simulink model "new_nncontroller_5_50"  (R2021a)
settings: Solver=VariableStepAuto  StartTime=0.0  StopTime=10.0  RelTol=1e-3
libraries: neural x257
(part 14 of 14)

== system new_nncontroller_5_50/Feed-Forward Neural Network/Layer 6/Delays 1 ==
  "p{6}" : Inport  PortDimensions=50
      mask Display: e = 0.06;c1 = [120 230 180]/255;c2 = ([120 230 180]+0)/(256+128);c3 = ([120 230 180]+128)/(256+128);patch([0 1 1 0],[0 0 1 1],c1);patch([0 1 1 1-e 1-e 0+e],[0 0 1 1-e 0+e 0+e],c2);patch([0 0 1 1-e 0+e 0+e],[0 1 1 1-e 1-e 0+e],c3);plot([0 1 1 0 0],[0 0 1 1 0]);
  mux : Mux  Inputs=1
      mask Display: e = 0.06;c1 = [120 150 230]/255;c2 = ([120 150 230]+0)/383;c3 = ([120 150 230]+128)/383;patch([0 1 1 0],[0 0 1 1],c1);patch([0 1 1 1-e 1-e 0+e],[0 0 1 1-e 0+e 0+e],c2);patch([0 0 1 1-e 0+e 0+e],[0 1 1 1-e 1-e 0+e],c3);plot([0 1 1 0 0],[0 0 1 1 0]);disp('Mux')
  "pd{6,5}" : Outport
      mask Display: e = 0.06;c1 = [120 230 180]/255;c2 = ([120 230 180]+0)/(256+128);c3 = ([120 230 180]+128)/(256+128);patch([0 1 1 0],[0 0 1 1],c1);patch([0 1 1 1-e 1-e 0+e],[0 0 1 1-e 0+e 0+e],c2);patch([0 0 1 1-e 0+e 0+e],[0 1 1 1-e 1-e 0+e],c3);plot([0 1 1 0 0],[0 0 1 1 0]);
  wires:
  "p{6}"/1 -> mux/1
  mux/1 -> "pd{6,5}"/1

== system new_nncontroller_5_50/Feed-Forward Neural Network/Layer 6/LW{6,5} ==
  "ad{6,5}" : Inport  PortDimensions=50
      mask Display: e = 0.06;c1 = [120 230 180]/255;c2 = ([120 230 180]+0)/(256+128);c3 = ([120 230 180]+128)/(256+128);patch([0 1 1 0],[0 0 1 1],c1);patch([0 1 1 1-e 1-e 0+e],[0 0 1 1-e 0+e 0+e],c2);patch([0 0 1 1-e 0+e 0+e],[0 1 1 1-e 1-e 0+e],c3);plot([0 1 1 0 0],[0 0 1 1 0]);
  "IW{6,5}(1,:)'" : Constant  Value=[0.7979373898433161915733080604695715010166168212890625;0.6425479901583213138138717113179154694080352783203125;0.953626015447462282992319160257466137409210205078125;0.16456963135197444358936991193331778049468994140625;-0.7833557479872637063778029187233187258243560791015625;0.84641809093803888064400098301121033728122711181640625;-0.452678124857251784618483725353144109249114990234375;-0.4806417329991887754658819176256656646728515625;0.483192247735164670530139119364321231842041015625;-0.11214184530773518844171121600084006786346435546875;-0.07122644724497136092811189200801891274750232696533203125;-0.328836955931493424287737070699222385883331298828125;0.37176760378130502271432078487123362720012664794921875;0.50256039224656234853938485684921033680438995361328125;-0.44622539087750789921216210132115520536899566650390625;0.7299507574428589773418707409291528165340423583984375;0.63513061455329589133356193997315131127834320068359375;-0.480777336847858283164214299176819622516632080078125;-0.80089327285409372958469020886695943772792816162109375;0.99338891001710660777490602413308806717395782470703125;-0.165296568054618620013940244461991824209690093994140625;-0.95196254834817406464964051338029094040393829345703125;-0.843578940168078883488078645314089953899383544921875;-0.406438626818008241770030508632771670818328857421875;-0.2108698573029774703257999135530553758144378662109375;-0.43149269314939975306089081641403026878833770751953125;-0.3923271110987835985639549107872880995273590087890625;0.65635842341370231878272534231655299663543701171875;0.8371619330413364590270930420956574380397796630859375;0.2003458956068105700776271760332747362554073333740234375;0.6483006783219626978365113245672546327114105224609375;0.9559537189805642487527848061290569603443145751953125;0.89602950292263272569215359908412210643291473388671875;0.3864724569906499151983325646142475306987762451171875;0.7390728395431003239224310163990594446659088134765625;0.72165942172722108427507237138343043625354766845703125;0.8675158384540109235416593946865759789943695068359375;-0.96125700373655298403008373497868888080120086669921875;0.0856695977515015416603461062550195492804050445556640625;0.77269072406629657479015804710797965526580810546875;0.307030128127842860674689973166096024215221405029296875;-0.5003409775365554867931905391742475330829620361328125;0.8958872248952542971522916559479199349880218505859375;-0.32479967997751824082541816096636466681957244873046875;-0.48588749013030019252568081356002949178218841552734375;0.5936172462406299477066795589053072035312652587890625;0.64434886072423136482711925054900348186492919921875;0.1118697655014558034469729363991064019501209259033203125;0.7034516827035119934663498497684486210346221923828125;-0.49219641359923926859920584320207126438617706298828125]
      mask Display: e = 0.06;c1 = [120 150 230]/255;c2 = ([120 150 230]+0)/383;c3 = ([120 150 230]+128)/383;patch([0 1 1 0],[0 0 1 1],c1);patch([0 1 1 1-e 1-e 0+e],[0 0 1 1-e 0+e 0+e],c2);patch([0 0 1 1-e 0+e 0+e],[0 1 1 1-e 1-e 0+e],c3);plot([0 1 1 0 0],[0 0 1 1 0]);disp('weights');
  Mux : Mux  Inputs=1
      mask Display: e = 0.06;c1 = [120 150 230]/255;c2 = ([120 150 230]+0)/383;c3 = ([120 150 230]+128)/383;patch([0 1 1 0],[0 0 1 1],c1);patch([0 1 1 1-e 1-e 0+e],[0 0 1 1-e 0+e 0+e],c2);patch([0 0 1 1-e 0+e 0+e],[0 1 1 1-e 1-e 0+e],c3);plot([0 1 1 0 0],[0 0 1 1 0]);disp('Mux');
  dotprod1 : neural/Weight Functions/dotprod
  "lz{6,5}" : Outport
      mask Display: e = 0.06;c1 = [120 230 180]/255;c2 = ([120 230 180]+0)/(256+128);c3 = ([120 230 180]+128)/(256+128);patch([0 1 1 0],[0 0 1 1],c1);patch([0 1 1 1-e 1-e 0+e],[0 0 1 1-e 0+e 0+e],c2);patch([0 0 1 1-e 0+e 0+e],[0 1 1 1-e 1-e 0+e],c3);plot([0 1 1 0 0],[0 0 1 1 0]);
  wires:
  "IW{6,5}(1,:)'"/1 -> dotprod1/1
  "ad{6,5}"/1 -> dotprod1/2
  dotprod1/1 -> Mux/1
  Mux/1 -> "lz{6,5}"/1
